simulink model "MotorGearRackTest"  (R2025a)
settings: Solver=ode15s  StartTime=0.0  StopTime=0.01  RelTol=1e-3
settings Model: Creator=Глеб  LastModifiedBy=Глеб

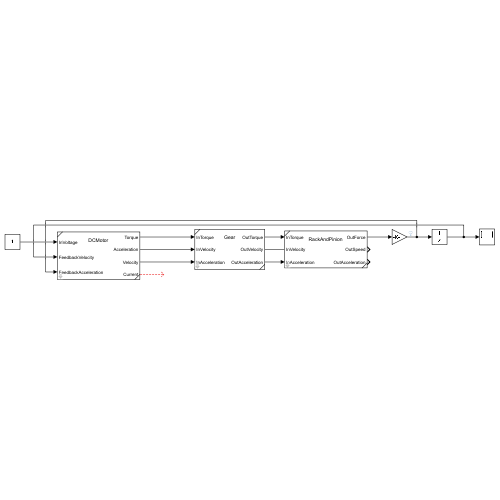
[thumbnail: Simulink's stored preview of the top-level diagram]
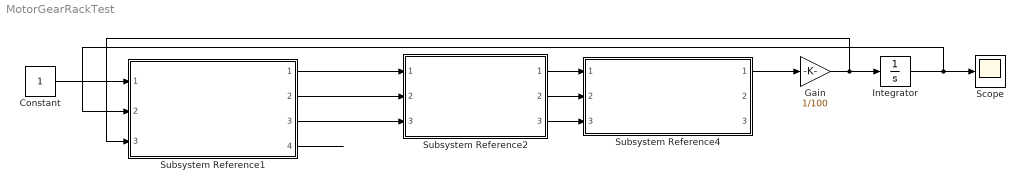
== system MotorGearRackTest ==
  Constant : Constant
  Gain : Gain  Gain=1/100
  Integrator : Integrator
  Scope : Scope
      settings: ActiveDisplayYMinimum=-0.036211036494644855  ActiveDisplayYMaximum=0.053369021624233737
  Subsystem Reference1 : Subsystem  ReferencedSubsystem=DCMotor  kw=60  L=350*10^-6  R=10  km=16  J_motor=500*10^-9  vis_friction_coef_motor=0.1
  Subsystem Reference2 : Subsystem  ReferencedSubsystem=Gear  i_gear=100  J_gear=2.4*10^-6  vis_friction_coef_gear=0.1
  Subsystem Reference4 : Subsystem  ReferencedSubsystem=RackAndPinion  i_coef=20  J_pinion=1*10^-6  m_rack=1  vis_friction_coef_rack=0.1
  wires:
  Constant/1 -> Subsystem Reference1/1
  Subsystem Reference1/1 -> Subsystem Reference2/1
  Subsystem Reference1/2 -> Subsystem Reference2/2
  Subsystem Reference1/3 -> Subsystem Reference2/3
  Subsystem Reference1/4 -> ?
  Subsystem Reference2/1 -> Subsystem Reference4/1
  Subsystem Reference2/2 -> Subsystem Reference4/2
  Subsystem Reference2/3 -> Subsystem Reference4/3
  Subsystem Reference4/1 -> Gain/1
  Gain/1 -> Subsystem Reference1/3, Integrator/1
  Integrator/1 -> Subsystem Reference1/2, Scope/1
